simulink model "lab4_2"  (R2021b)
settings: Solver=VariableStepAuto  StartTime=0.0  StopTime=10.0  RelTol=1e-3
values from neighbouring files (symbols this model uses):
  a = 0.8109    [s2_1.m]    (also in s2_2.m; s2_3.m)
  b = 6.575    [s2_1.m]    (also in s2_2.m; s2_3.m)
  K = rlocfind(G)    [s2_1.m]    (also in s2_2.m; s2_3.m)
  theta = 0    [s2_2.m]    (also in s2_3.m)
  Ti = TI    (= 0.0835625)    [s2_2.m]    (also in s2_3.m = 0.059361)
  VMAX_UPM = 11.75    [s2_2.m]    (also in s2_3.m)
settings Model: Creator=adanm  LastModifiedBy=Juho
settings SolverCC: AlgebraicLoopSolver=TrustRegion
settings DataIOCC: ReturnWorkspaceOutputs=off
settings DebuggingCC: SFMachineParentedDataDiag=warning  ArithmeticOperatorsInVariantConditions=warning
settings SFSimCC: CustomCodeUndefinedFunction=UseInterfaceOnly

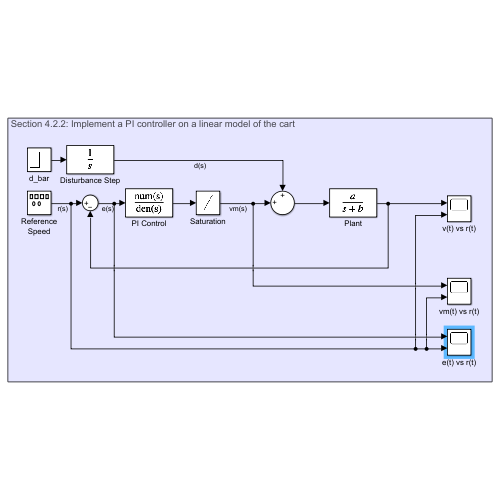
[thumbnail: Simulink's stored preview of the top-level diagram]
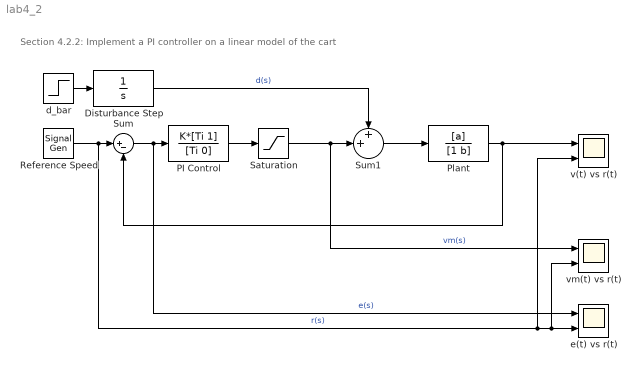
== system lab4_2 ==
  note: Section 4.2.2: Implement a PI controller on a linear model of the cart
  Disturbance Step : TransferFcn  Denominator=[1 0]
  PI Control : TransferFcn  Numerator=K*[Ti 1]  Denominator=[Ti 0]
  Plant : TransferFcn  Numerator=[a]  Denominator=[1 b]
  Reference Speed : SignalGenerator  WaveForm=square  Amplitude=0.2  Frequency=0.5
  "Saturation " : Saturate  UpperLimit=VMAX_UPM  LowerLimit=-VMAX_UPM
  Sum : Sum  Inputs=|+-
  Sum1 : Sum  Inputs=++|
  d_bar : Step  Time=0  After=9.81*sin(theta)/a  SampleTime=0
  e(t) vs r(t) : Scope  NumInputPorts=2
  v(t) vs r(t) : Scope  NumInputPorts=2
  vm(t) vs r(t) : Scope  NumInputPorts=2
  wires:
  Reference Speed/1 -> v(t) vs r(t)/2, vm(t) vs r(t)/2, e(t) vs r(t)/2, Sum/1  "r(s)"
  d_bar/1 -> Disturbance Step/1
  Sum1/1 -> Plant/1
  Disturbance Step/1 -> Sum1/1  "d(s)"
  Sum/1 -> e(t) vs r(t)/1, PI Control/1  "e(s)"
  Plant/1 -> v(t) vs r(t)/1, Sum/2
  PI Control/1 -> "Saturation "/1
  "Saturation "/1 -> vm(t) vs r(t)/1, Sum1/2  "vm(s)"
